simulink model "bb2_vertical_linear_tracking"  (R2025a)
settings: Solver=VariableStepAuto  StartTime=0.0  StopTime=350  RelTol=1e-3
values from neighbouring files (symbols this model uses):
  A = [ -9.6e-13  5.0e+00   1.0e+00   1.1e-10 ... (first row only)    [setup_bb2_vertical.m]
  Bv = B(:,1)    [setup_bb2_vertical.m]
  Cout = [C; eye(4)]    [setup_bb2_vertical.m]
  Dout = [0; zeros(4,1)]    [setup_bb2_vertical.m]
  Keta = Kz(:, 5:end)    [setup_bb2_vertical.m]
  Kx = Kz(:, 1:4)    [setup_bb2_vertical.m]
  r_points = [-100 -100 -50 -30]    [setup_bb2_vertical.m]
  S = [0 1 0 0 ... (first row only)    [setup_bb2_vertical.m]
  Tf = 200    [setup_bb2_vertical.m]
  Upsilon = [0;0;0;1]    [setup_bb2_vertical.m]
settings Model: Creator=mohammad  LastModifiedBy=mohammadghavidelvahid

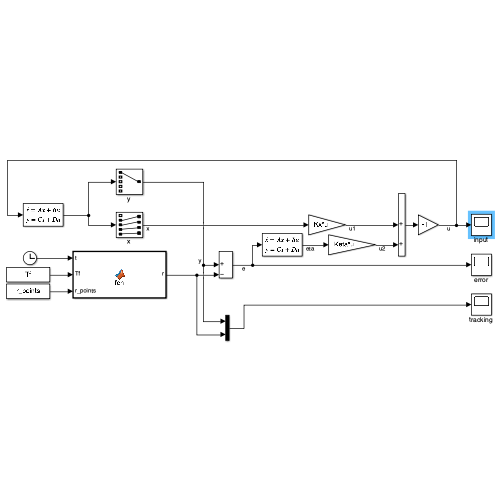
[thumbnail: Simulink's stored preview of the top-level diagram]
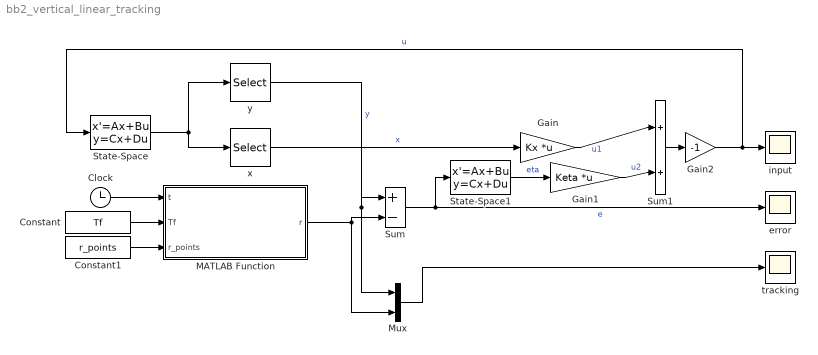
== system bb2_vertical_linear_tracking ==
  Clock : Clock
  Constant : Constant  Value=Tf
  Constant1 : Constant  Value=r_points
  Gain : Gain  Gain=Kx  Multiplication=Matrix(K*u)
  Gain1 : Gain  Gain=Keta  Multiplication=Matrix(K*u)
  Gain2 : Gain  Gain=-1
  MATLAB Function : MATLAB Function  TreatAsAtomicUnit=on
  Mux : Mux  Inputs=2
  State-Space : StateSpace  A=A  B=Bv  C=Cout  D=Dout  InitialCondition=[-100; 0; 0; 0]
  State-Space1 : StateSpace  A=S  B=Upsilon  C=eye(4)  D=zeros(4,1)  InitialCondition=zeros(4,1)
  Sum : Sum  Inputs=|+-
  Sum1 : Sum  Inputs=|++
  error : Scope
      settings: ActiveDisplayYMinimum=-747.56840198460793  ActiveDisplayYMaximum=681.55733426592906
  input : Scope
      settings: ActiveDisplayYMinimum=-1316.7889279664673  ActiveDisplayYMaximum=2869.2181956068553  DataLoggingVariableName=ScopeData2
  tracking : Scope
      settings: ActiveDisplayYMinimum=-1410.2270978580345  ActiveDisplayYMaximum=373.75693626153372  DataLoggingVariableName=ScopeData3
  x : Selector  InputPortWidth=5  IndexOptions=Index vector (dialog)  Indices=2:5  OutputSizes=1
  y : Selector  InputPortWidth=5  IndexOptions=Index vector (dialog)  Indices=1  OutputSizes=1
  wires:
  State-Space/1 -> x/1, y/1
  Sum/1 -> error/1, State-Space1/1  "e"
  State-Space1/1 -> Gain1/1  "eta"
  y/1 -> Mux/1, Sum/1  "y"
  Gain/1 -> Sum1/1  "u1"
  Gain1/1 -> Sum1/2  "u2"
  Sum1/1 -> Gain2/1
  Mux/1 -> tracking/1
  x/1 -> Gain/1  "x"
  Gain2/1 -> State-Space/1, input/1  "u"
  MATLAB Function/1(r) -> Mux/2, Sum/2
  Clock/1 -> MATLAB Function/1(t)
  Constant/1 -> MATLAB Function/2(Tf)
  Constant1/1 -> MATLAB Function/3(r_points)

== matlab function bb2_vertical_linear_tracking/MATLAB Function ==
  data: t input; r output; Tf input; r_points input
function r = fcn(t, Tf, r_points)
r = bernstein_ref(t, Tf, r_points);
end
